simulink model "Servomotor_Complete"  (Simulink 7.2)
settings: Solver=ode23t  StartTime=0.0  StopTime=5  FixedStep=0.001  MaxStep=0.1  RelTol=10e-3
libraries: mblibv1 x10, fl_lib x5, nesl_utility x2, simulink x1, elec_lib x1, dsparch4 x1
settings Model: Creator=LAraujo  LastModifiedBy=LAraujo
settings SolverCC: SolverResetMethod=Robust
settings SimMechanicsCC: VisDuringSimulation=on

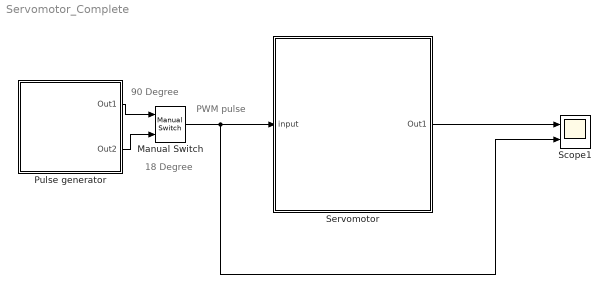
== system Servomotor_Complete ==
  note: PWM pulse
  note: 90 Degree
  note: 18 Degree
  Manual Switch : simulink/Signal Routing/Manual Switch  SystemSampleTime=-1  sw=1  action=0  varsize=off
  Pulse generator : Subsystem
      mask Display: image(imread('PulseGen.JPG'))
  Scope1 : Scope  NumInputPorts=2
      settings: TimeRange=0.5  YMin=-60~0  YMax=0~1
  Servomotor : Subsystem
      mask Display: image(imread('spe_servomotor_motor.jpg'))
  wires:
  Manual Switch/1 -> Servomotor/1(input), Scope1/2
  Pulse generator/1(Out1) -> Manual Switch/1
  Pulse generator/2(Out2) -> Manual Switch/2
  Servomotor/1(Out1) -> Scope1/1

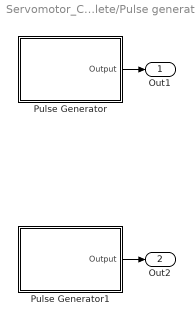
== system Servomotor_Complete/Pulse generator ==
  Pulse Generator : Subsystem  mask{Pulse=1.5}
      mask prompts: Pulse "Pulse width"
  Pulse Generator1 : Subsystem  mask{Pulse=1.3}
      mask prompts: Pulse "Pulse width"
  Out1 : Outport
  Out2 : Outport  Port=2
  wires:
  Pulse Generator/1(Output) -> Out1/1
  Pulse Generator1/1(Output) -> Out2/1

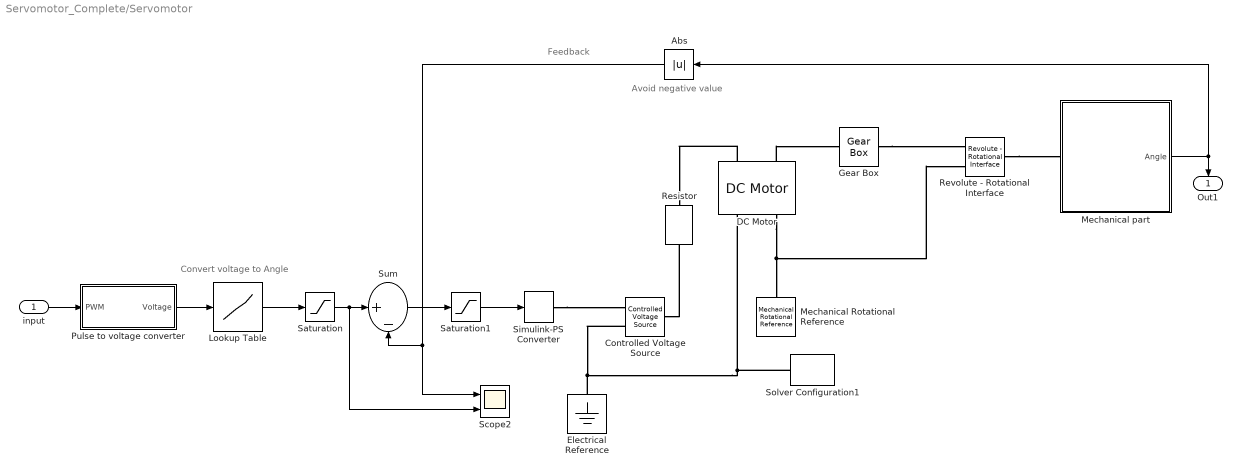
== system Servomotor_Complete/Servomotor ==
  note: Convert voltage to Angle
  note: Avoid negative value
  note: Feedback
  input : Inport
  Abs : Abs  Orientation=left  OutDataType=sfix(16)  OutScaling=2^0
  Controlled Voltage Source : fl_lib/Electrical/Electrical Sources/Controlled Voltage Source  Orientation=left  DialogController=NetworkEngine.DynNeDlgSource  SystemSampleTime=-1  current_Log=off  voltage_Log=off  power_Log=off  LocalVarNames=|current|voltage|power  LocalVarDescs=|Current (A)|Voltage (V)|Power (W)  LocalVarLogging=[0 0 0]
  DC Motor : elec_lib/Actuators & Drivers/DC Motor  Orientation=down  DialogController=NetworkEngine.DynNeDlgSource  SystemSampleTime=-1  parameterization=1  Ra=10 Ohm  La=1.2e-08 H  emf_or_torque=1  Kv=7.2e-05 V/rpm  Ki=6.876e-04 N*m/A  T_stall=2.4e-04 N*m  w_max=1.91e+04 rpm  w_rated=1.5e+04 rpm  P_rated=0.08 W  V_rated=1.5 V  J=0 g*cm^2  lam=1e-06 N*m/(rad/s)  speed0=0 rpm  current_Log=off  voltage_Log=off  power_Log=off  i2r_Log=off  torque_Log=off  speed_Log=off  LocalVarNames=|current|voltage|power|i2r|torque|speed  LocalVarDescs=|Current (A)|Voltage (V)|Power (W)|Electrical losses (W)|Torque (Nm)|Angular speed (rad/s)  LocalVarLogging=[0 0 0 0 0 0]
  Electrical Reference : fl_lib/Electrical/Electrical Elements/Electrical Reference  Orientation=down  DialogController=NetworkEngine.DynNeDlgSource  SystemSampleTime=-1  LocalVarLogging=[]
  Gear Box : fl_lib/Mechanical/Mechanisms/Gear Box  DialogController=NetworkEngine.DynNeDlgSource  SystemSampleTime=-1  ratio=5  torque_inp_Log=off  ang_velocity_inp_Log=off  power_Log=off  LocalVarNames=|torque_inp|ang_velocity_inp|power  LocalVarDescs=|Input shaft torque (N*m)|Input shaft angular velocity (rad/s)|Power transmitted by the box (W)  LocalVarLogging=[0 0 0]
  Lookup Table : Lookup  InputValues=[62.51,75.01,87.51]  Table=[0,90,180]  OutDataType=sfix(16)  OutScaling=2^0
  Mechanical Rotational Reference : fl_lib/Mechanical/Rotational Elements/Mechanical Rotational Reference  Orientation=down  DialogController=NetworkEngine.DynNeDlgSource  SystemSampleTime=-1  LocalVarLogging=[]
  Mechanical part : Subsystem
      mask Display: image(imread('hitec_servo_b.jpg'))
  Pulse to voltage converter : Subsystem
  Resistor : fl_lib/Electrical/Electrical Elements/Resistor  Orientation=down  DialogController=NetworkEngine.DynNeDlgSource  SystemSampleTime=-1  R=50 Ohm  current_Log=off  voltage_Log=off  power_Log=off  LocalVarNames=|current|voltage|power  LocalVarDescs=|Resistor current (A)|Voltage across resistor (V)|Power (W)  LocalVarLogging=[0 0 0]
  Revolute - Rotational Interface : mblibv1/Interface  Elements/Revolute - Rotational Interface  DialogController=MECH.DynMechDlgSource  SystemSampleTime=-1  UpdateFromCAD=off  DialogClass=RevoluteRotationalInterface  Primitive=R1
  Saturation : Saturate  UpperLimit=180  LowerLimit=0  LinearizeAsGain=off  ZeroCross=off  OutDataType=sfix(16)  OutScaling=2^0
  Saturation1 : Saturate  UpperLimit=70  LowerLimit=-70  LinearizeAsGain=off  ZeroCross=off  OutDataType=sfix(16)  OutScaling=2^0
  Scope2 : Scope  NumInputPorts=2
      settings: YMin=0~0  YMax=100~100  SaveName=ScopeData2
  Simulink-PS Converter : nesl_utility/Simulink-PS Converter  DialogController=NetworkEngine.DynNeUtilDlgSource  SystemSampleTime=-1  PhysicalDomain=network_engine_domain  LeftPortType=input  RightPortType=output  SubClassName=ps_input  Unit=1  AffineConversion=off  InputFilterTimeConstant=.001  UdotUserProvided=0
  Solver Configuration1 : nesl_utility/Solver Configuration  Orientation=left  DialogController=NetworkEngine.DynNeUtilDlgSource  SystemSampleTime=-1  PhysicalDomain=network_engine_domain  LeftPortType=input  RightPortType=generic  SubClassName=solver  Accelerate=off  Profile=off  ResidualTolerance=1e-9  MaxNonlinIter=12  MaxModeIter=2  DoFixedCost=off  DoDC=off  LinearAlgebra=Sparse
  Sum : Sum  Inputs=|+-  OutDataType=sfix(16)  OutScaling=2^0
  Out1 : Outport  Orientation=down
  wires:
  Mechanical part/1(Angle) -> Abs/1, Out1/1
  Pulse to voltage converter/1(Voltage) -> Lookup Table/1
  Lookup Table/1 -> Saturation/1
  Saturation/1 -> Sum/1, Scope2/2
  Sum/1 -> Saturation1/1
  Saturation1/1 -> Simulink-PS Converter/1
  Abs/1 -> Sum/2, Scope2/1
  input/1 -> Pulse to voltage converter/1(PWM)
  connections:
  Controlled Voltage Source/LConn1 -- Resistor/RConn1
  Simulink-PS Converter/RConn1 -- Controlled Voltage Source/RConn1
  Controlled Voltage Source/RConn2 -- DC Motor/RConn1 -- Solver Configuration1/RConn1 -- Electrical Reference/LConn1
  DC Motor/LConn1 -- Resistor/LConn1
  DC Motor/LConn2 -- Gear Box/LConn1
  DC Motor/RConn2 -- Mechanical Rotational Reference/LConn1 -- Revolute - Rotational Interface/LConn2
  Gear Box/RConn1 -- Revolute - Rotational Interface/LConn1
  Revolute - Rotational Interface/RConn1 -- Mechanical part/LConn1

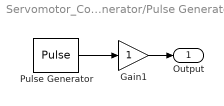
== system Servomotor_Complete/Pulse generator/Pulse Generator ==
  Gain1 : Gain  ParameterDataType=sfix(16)  ParameterScaling=2^0  OutDataType=sfix(16)  OutScaling=2^0
  Pulse Generator : DiscretePulseGenerator  PulseType=Time based  Period=20e-3  PulseWidth=(Pulse*100)/20
  Output : Outport
  wires:
  Pulse Generator/1 -> Gain1/1
  Gain1/1 -> Output/1

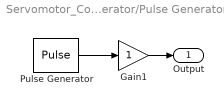
== system Servomotor_Complete/Pulse generator/Pulse Generator1 ==
  Gain1 : Gain  ParameterDataType=sfix(16)  ParameterScaling=2^0  OutDataType=sfix(16)  OutScaling=2^0
  Pulse Generator : DiscretePulseGenerator  PulseType=Time based  Period=20e-3  PulseWidth=(Pulse*100)/20
  Output : Outport
  wires:
  Pulse Generator/1 -> Gain1/1
  Gain1/1 -> Output/1

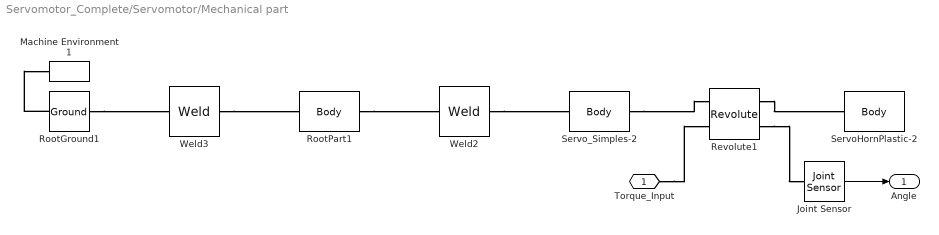
== system Servomotor_Complete/Servomotor/Mechanical part ==
  Joint Sensor : mblibv1/Sensors &  Actuators/Joint Sensor  DialogController=MECH.DynMechDlgSource  SystemSampleTime=-1  UpdateFromCAD=off  PhysicalDomain=Mechanical  PortType=blob  Muxed=on  Pose=off  Angle=on  AngleUnits=deg  ArcVelocity=off  ArcVelocityUnits=deg/s  ArcAcceleration=off  ArcAccelerationUnits=deg/s^2  CoordPosition=on  CoordPositionUnits=m  Velocity=off  VelocityUnits=m/s  Acceleration=off  AccelerationUnits=m/s^2  Quaternion=on  QuaternionDT=off  QuaternionDDT=off  QuaternionUnits=off  OutputVector=[1]  ActiveIO=on  Width=1  DialogClass=MechanicalSensorBlock  Primitive=R1  Force=off  ForceUnits=N  Torque=off  TorqueUnits=N*m  ReferenceFrame=Absolute (World)  ReactionSensedSide=Base  ReactionReferenceFrame=Absolute (World)  ReactionForce=off  ReactionForceUnits=N  ReactionMoment=off  ReactionMomentUnits=N*m
  Machine Environment1 : mblibv1/Bodies/Machine Environment  Orientation=left  DialogController=MECH.DialogSource  SystemSampleTime=-1  PortType=env  PhysicalDomain=Mechanical  DialogTemplateClass=MECH.MachineEnvironment  SyncWhenCopied=off  Gravity=[0 -9.81 0]  GravityUnits=m/s^2  GravityAsSignal=off  Dimensionality=Auto-detect  AnalysisType=Forward dynamics  LinearAssemblyTolerance=1e-3  LinearAssemblyToleranceUnits=m  AngularAssemblyTolerance=1e-3  AngularAssemblyToleranceUnits=rad  ConstraintSolverType=Stabilizing  ConstraintRelTolerance=1e-4  ConstraintAbsTolerance=1e-4  UseRobustSingularityHandling=off  RedundancyAnalysisToleranceType=Automatically select tolerance  RedundancyAnalysisTolerance=1e-14  StatePerturbationType=Fixed  PerturbationSize=1e-5  VisualizeMachine=on  BodyVisualizationType=Use model default body geometries  BodyColorSelMode=Use model default  DefaultBodyColor=[1 0 0]
  Revolute1 : mblibv1/Joints/Revolute  DialogController=MECH.DynMechDlgSource  PhysicalDomain=mechanical  SubClassName=Unknown  LeftPortType=blob  RightPortType=blob  LConnTagsString=__newl0|SA1  RConnTagsString=__newr0|SA1  UpdateFromCAD=on  NumSAPorts=2  CutJoint=off  MarkAsCut=off  Primitives=prismatic  PrimitiveProps=R1$World$[0,0,1]$revolute  DialogClass=JointBlock  R1Axis=[0,0,1]
  RootGround1 : mblibv1/Bodies/Ground  DialogController=MECH.DynMechDlgSource  SystemSampleTime=-1  UpdateFromCAD=on  LeftPortType=env  RightPortType=workingframe  PhysicalDomain=Mechanical  DialogClass=GroundBlock  CoordPosition=[-0.00325605,0.000392966,-0.00120744]  CoordPositionUnits=m  StateVectorMgrId=2  MachineId=[3 0]  ShowEnvPort=on
  RootPart1 : mblibv1/Bodies/Body  DialogController=MECH.DynMechDlgSource  PhysicalDomain=mechanical  SubClassName=Unknown  LeftPortType=workingframe  RightPortType=workingframe  LConnTagsString=CS3  RConnTagsString=CS2  UpdateFromCAD=on  DialogClass=MechanicalBodyBlock  Mass=0  MassUnits=kg  InertiaUnits=kg*m^2  Inertia=[0,0,0;0,0,0;0,0,0]  Shape=Cylinder  ShapeDims=[1 1]  ShapeUnits=m  ShapeUse=false  Density=1  DensityUnits=kg/m^3  DensityUse=false  GraphicsMode=MACHINE_DEFAULT  BodyColorSelMode=MACHINE_DEFAULT  BodyColor=[1 0 0]  AttachedToCS=CS1  CG=Right$CG$[-0.00325605 0.000392966 -0.00120744]$WORLD$WORLD$m$[1 0 0;0 1 0;0 0 1]$3x3 Transform$rad$WORLD$false$none  WorkingFrames=Right$CS1$[0 0 0]$WORLD$WORLD$m$[1 0 0;0 1 0;0 0 1]$3x3 Transform$rad$WORLD$false$none#Right$CS2$[-0.00331151 0.00039206 -0.00109331]$WORLD$WORLD$m$[1 0 0;0 1 0;0 0 1]$3x3 Transform$rad$WORLD$true$none#Left$CS3$[-0.00325605 0.000392966 -0.00120744]$WORLD$WORLD$m$[1 0 0;0 1 0;0 0 1]$3x3 Transform$rad$WORLD$true$none  CGPos=[-0.00325605 0.000392966 -0.00120744]  CGRot=[1 0 0;0 1 0;0 0 1]  CS0Pos=[]  CS0Rot=[]  CS1Pos=[0 0 0]  CS1Rot=[1 0 0;0 1 0;0 0 1]  CS2Pos=[-0.00331151 0.00039206 -0.00109331]  CS2Rot=[1 0 0;0 1 0;0 0 1]  CS3Pos=[-0.00325605 0.000392966 -0.00120744]  CS3Rot=[1 0 0;0 1 0;0 0 1]  CS4Pos=[]  CS4Rot=[]  CS5Pos=[]  CS5Rot=[]  CS6Pos=[]  CS6Rot=[]  CS7Pos=[]  CS7Rot=[]  CS8Pos=[]  CS8Rot=[]  CS9Pos=[]  CS9Rot=[]  CS10Pos=[]  CS10Rot=[]  CS11Pos=[]  CS11Rot=[]  CS12Pos=[]  CS12Rot=[]  CS13Pos=[]  CS13Rot=[]  CS14Pos=[]  CS14Rot=[]  CS15Pos=[]  CS15Rot=[]  CS16Pos=[]  CS16Rot=[]  CS17Pos=[]  CS17Rot=[]  CS18Pos=[]  CS18Rot=[]  CS19Pos=[]  CS19Rot=[]  CS20Pos=[]  CS20Rot=[]
  ServoHornPlastic-2 : mblibv1/Bodies/Body  DialogController=MECH.DynMechDlgSource  PhysicalDomain=mechanical  SubClassName=Unknown  LeftPortType=workingframe  RightPortType=workingframe  LConnTagsString=CS2  UpdateFromCAD=on  DialogClass=MechanicalBodyBlock  Mass=0.00107043  MassUnits=kg  InertiaUnits=kg*m^2  Inertia=[3.77224e-008,0,0;0,7.26212e-008,0;0,0,3.65964e-008]  Shape=Cylinder  ShapeDims=[1 1]  ShapeUnits=m  ShapeUse=false  Density=1  DensityUnits=kg/m^3  DensityUse=false  GraphicsMode=GFXFILE  GraphicsFileName=Montagem_ServoSimples - ServoHornPlastic-1.STL  BodyColorSelMode=COLORPALETTE  BodyColor=[0.698039;0.698039;0.698039]  AttachedToCS=CS1  CG=Right$CG$[0.00667762 0.000555315 -0.0216488]$WORLD$WORLD$m$[0.999756 0 -0.0220735;0.0220735 0 0.999756;0 -1 0]$3x3 Transform$rad$WORLD$false$none  WorkingFrames=Right$CS1$[0.00667762 0.000555315 -0.02285]$WORLD$WORLD$m$[0.999756 0 -0.0220735;0.0220735 0 0.999756;0 -1 0]$3x3 Transform$rad$WORLD$false$none#Left$CS2$[0.00667762 0.000555315 -0.02135]$WORLD$WORLD$m$[1 0 0;0 1 0;0 0 1]$3x3 Transform$rad$WORLD$true$none  CGPos=[0.00667762 0.000555315 -0.0216488]  CGRot=[0.999756 0 -0.0220735;0.0220735 0 0.999756;0 -1 0]  CS0Pos=[]  CS0Rot=[]  CS1Pos=[0.00667762 0.000555315 -0.02285]  CS1Rot=[0.999756 0 -0.0220735;0.0220735 0 0.999756;0 -1 0]  CS2Pos=[0.00667762 0.000555315 -0.02135]  CS2Rot=[1 0 0;0 1 0;0 0 1]  CS3Pos=[]  CS3Rot=[]  CS4Pos=[]  CS4Rot=[]  CS5Pos=[]  CS5Rot=[]  CS6Pos=[]  CS6Rot=[]  CS7Pos=[]  CS7Rot=[]  CS8Pos=[]  CS8Rot=[]  CS9Pos=[]  CS9Rot=[]  CS10Pos=[]  CS10Rot=[]  CS11Pos=[]  CS11Rot=[]  CS12Pos=[]  CS12Rot=[]  CS13Pos=[]  CS13Rot=[]  CS14Pos=[]  CS14Rot=[]  CS15Pos=[]  CS15Rot=[]  CS16Pos=[]  CS16Rot=[]  CS17Pos=[]  CS17Rot=[]  CS18Pos=[]  CS18Rot=[]  CS19Pos=[]  CS19Rot=[]  CS20Pos=[]  CS20Rot=[]
  Servo_Simples-2 : mblibv1/Bodies/Body  DialogController=MECH.DynMechDlgSource  PhysicalDomain=mechanical  SubClassName=Unknown  LeftPortType=workingframe  RightPortType=workingframe  LConnTagsString=CS2  RConnTagsString=CS3  UpdateFromCAD=on  DialogClass=MechanicalBodyBlock  Mass=0.191711  MassUnits=kg  InertiaUnits=kg*m^2  Inertia=[2.66902e-005,-2.21506e-009,-3.18594e-007;-2.21506e-009,4.55319e-005,9.87505e-009;-3.18594e-007,9.87505e-009,3.14869e-005]  Shape=Cylinder  ShapeDims=[1 1]  ShapeUnits=m  ShapeUse=false  Density=1  DensityUnits=kg/m^3  DensityUse=false  GraphicsMode=GFXFILE  GraphicsFileName=Montagem_ServoSimples - Servo_Simples-1.STL  BodyColorSelMode=COLORPALETTE  BodyColor=[0.231373;0.231373;0.231373]  AttachedToCS=CS1  CG=Right$CG$[-0.00331151 0.00039206 -0.00109331]$WORLD$WORLD$m$[1 0 0;0 1 0;0 0 1]$3x3 Transform$rad$WORLD$false$none  WorkingFrames=Right$CS1$[0.00672906 -0.00941128 -1.65475e-014]$WORLD$WORLD$m$[1 0 0;0 1 0;0 0 1]$3x3 Transform$rad$WORLD$false$none#Left$CS2$[-0.00331151 0.00039206 -0.00109331]$WORLD$WORLD$m$[1 0 0;0 1 0;0 0 1]$3x3 Transform$rad$WORLD$true$none#Right$CS3$[0.00667762 0.000555315 -0.02135]$WORLD$WORLD$m$[1 0 0;0 1 0;0 0 1]$3x3 Transform$rad$WORLD$true$none  CGPos=[-0.00331151 0.00039206 -0.00109331]  CGRot=[1 0 0;0 1 0;0 0 1]  CS0Pos=[]  CS0Rot=[]  CS1Pos=[0.00672906 -0.00941128 -1.65475e-014]  CS1Rot=[1 0 0;0 1 0;0 0 1]  CS2Pos=[-0.00331151 0.00039206 -0.00109331]  CS2Rot=[1 0 0;0 1 0;0 0 1]  CS3Pos=[0.00667762 0.000555315 -0.02135]  CS3Rot=[1 0 0;0 1 0;0 0 1]  CS4Pos=[]  CS4Rot=[]  CS5Pos=[]  CS5Rot=[]  CS6Pos=[]  CS6Rot=[]  CS7Pos=[]  CS7Rot=[]  CS8Pos=[]  CS8Rot=[]  CS9Pos=[]  CS9Rot=[]  CS10Pos=[]  CS10Rot=[]  CS11Pos=[]  CS11Rot=[]  CS12Pos=[]  CS12Rot=[]  CS13Pos=[]  CS13Rot=[]  CS14Pos=[]  CS14Rot=[]  CS15Pos=[]  CS15Rot=[]  CS16Pos=[]  CS16Rot=[]  CS17Pos=[]  CS17Rot=[]  CS18Pos=[]  CS18Rot=[]  CS19Pos=[]  CS19Rot=[]  CS20Pos=[]  CS20Rot=[]
  Weld2 : mblibv1/Joints/Weld  DialogController=MECH.DynMechDlgSource  PhysicalDomain=mechanical  SubClassName=Unknown  LeftPortType=blob  RightPortType=blob  LConnTagsString=__newl0  RConnTagsString=__newr0  UpdateFromCAD=on  NumSAPorts=0  CutJoint=off  MarkAsCut=off  Primitives=weld  PrimitiveProps=W$WORLD$[0.57735,0.57735,0.57735]$weld  DialogClass=JointBlock  WAxis=[0.57735,0.57735,0.57735]
  Weld3 : mblibv1/Joints/Weld  DialogController=MECH.DynMechDlgSource  PhysicalDomain=mechanical  SubClassName=Unknown  LeftPortType=blob  RightPortType=blob  LConnTagsString=__newl0  RConnTagsString=__newr0  UpdateFromCAD=on  NumSAPorts=0  CutJoint=off  MarkAsCut=off  Primitives=weld  PrimitiveProps=W$WORLD$[0.57735,0.57735,0.57735]$weld  DialogClass=JointBlock  WAxis=[0.57735,0.57735,0.57735]
  Torque_Input : PMIOPort  Port=1  Side=Left
  Angle : Outport  OutDataType=sfix(16)  OutScaling=2^0
  wires:
  Joint Sensor/1 -> Angle/1
  connections:
  RootPart1/RConn1 -- Weld2/LConn1
  Weld2/RConn1 -- Servo_Simples-2/LConn1
  Servo_Simples-2/RConn1 -- Revolute1/LConn1
  Revolute1/RConn1 -- ServoHornPlastic-2/LConn1
  RootGround1/RConn1 -- Weld3/LConn1
  Weld3/RConn1 -- RootPart1/LConn1
  RootGround1/LConn1 -- Machine Environment1/RConn1
  Torque_Input/RConn1 -- Revolute1/LConn2
  Revolute1/RConn2 -- Joint Sensor/LConn1

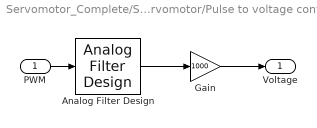
== system Servomotor_Complete/Servomotor/Pulse to voltage converter ==
  PWM : Inport
  Analog Filter Design : dsparch4/Analog Filter Design  method=Bessel  filttype=Lowpass  N=5  Wlo=50  Whi=80  Rp=2  Rs=40
  Gain : Gain  Gain=1000  ParameterDataType=sfix(16)  ParameterScaling=2^0  OutDataType=sfix(16)  OutScaling=2^0
  Voltage : Outport
  wires:
  Analog Filter Design/1 -> Gain/1
  PWM/1 -> Analog Filter Design/1
  Gain/1 -> Voltage/1
